simulink model "MP_TX"  (R2021a)
settings: Solver=VariableStepAuto  StartTime=0.0  StopTime=100000  RelTol=1e-3
undefined symbols (not defined in the file): Fs, ip, usb
libraries: plutoradiolib x1, audiosources x1, commanabbnd3 x1
settings Model: Creator=nitis  LastModifiedBy=nitis

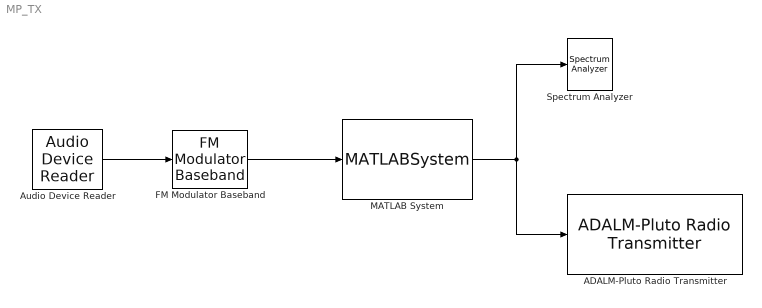
== system MP_TX ==
  ADALM-Pluto Radio Transmitter : plutoradiolib/ADALM-Pluto Radio Transmitter  RadioID=usb:0  uri=ip:10.0.0.200  CenterFrequencySource=Dialog  CenterFrequency=433e6  GainSource=Dialog  Gain=-10  ChannelMapping=1  BasebandSampleRate=192e3  UnderflowOutputPort=off  ShowAdvancedProperties=off  UseCustomFilter=off  filtPathRates=[737280000 11520000 3840000 1920000 960000 240000]  filtCoefficients=[-192 82 85 -215 228 -102 -110 290 -318 145 160 -426 471 -215 -238 633 -697 318 349 -923 1009 -457 -498 1309 -1423 640 693 -1812 1959 -876 -945 2458 -2647 1180 1268 -3290 3534 -1572 -1688 4375 -4698 2091 2247 -5836 6284 -2807 -3031 7918 -8588 3870 4225 -11182 12324 -5662 -6330 17255 -19735 9507 11312 -33568 43355 -25227 -42139 305542 305542 -42139 -25227 43355 -33568 11312 9507 -19735 17255 -6330 -5662 12324 -11182 4225 3870 -8588 7918 -3031 -2807 6284 -5836 2247 2091 -4698 4375 -1688 -1572 3534 -3290 1268 1180 -2647 2458 -945 -876 1959 -1812 693 640 -1423 1309 -498 -457 1009 -923 349 318 -697 633 -238 -215 471 -426 160 145 -318 290 -110 -102 228 -215 85 82 -192]  filtCoefficientSize=128  filtDecimInterpFactor=4  filtGain=-12  filtRFBandwidth=18000000  filterConfigStruct=struct()  DataSourceSelect=Input Port  DDSTone1Freq=5e3  DDSTone2Freq=10e3  DDSTone1Scale=0.5  DDSTone2Scale=0.25  DataTimeout=Inf  FrequencyCorrection=0  ENSMPinControlMode=None  BISTLoopbackMode=Disabled  BISTToneInject=Disabled  BISTSignalGen=PRBS  BISTToneFreq=Fs/32  BISTToneLevel=0
      settings: SourceProductBaseCode=PLUTO
  Audio Device Reader : audiosources/Audio Device Reader  Driver=DirectSound  Device=Default  SampleRate=192e3  NumChannels=1  SamplesPerFrame=20000  BitDepth=16-bit integer  NumBuffers=10  DefaultInputChannelMapping=on  InputChannelMapping=1:2  OutputNumOverrunSamples=off  OutputDataType=double  DriverIdx=1  DeviceWarnFlag=''
      settings: SourceProductBaseCode=AU
  FM Modulator Baseband : commanabbnd3/FM Modulator Baseband  FrequencyDeviation=75e3  SimulateUsing=Code generation
      settings: SourceProductBaseCode=CM
  MATLAB System : MATLABSystem  System=PlutoFMTransmit  SampleRate=192e3  SimulateUsing=Code generation
      mask Type: PlutoFMTransmit
      mask Display:
      | disp('PlutoFMTransmit');
      | port_label('input',1,'u');
      | port_label('output',1,'y');
  Spectrum Analyzer : SpectrumAnalyzer
  wires:
  Audio Device Reader/1 -> FM Modulator Baseband/1
  FM Modulator Baseband/1 -> MATLAB System/1
  MATLAB System/1 -> ADALM-Pluto Radio Transmitter/1, Spectrum Analyzer/1
